simulink subsystem "OperatingModeAndErrorLogic"  (R2023b)
settings: Solver=VariableStepAuto  StartTime=0.0  StopTime=10  RelTol=1e-3
undefined symbols (not defined in the file): operatingMode
libraries: simulink x2
settings Model: DefaultTestHarness=Supervisory_Logic_Harness  Creator=vlenzi  LastModifiedBy=vlenzi

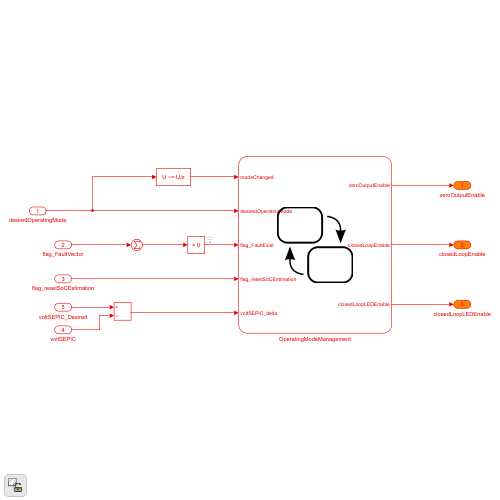
[thumbnail: Simulink's stored preview of the top-level diagram]
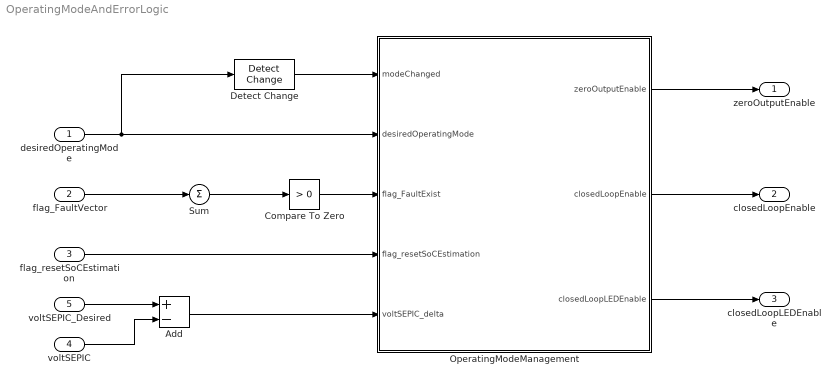
== system OperatingModeAndErrorLogic ==
  desiredOperatingMode : Inport
  flag_FaultVector : Inport  Port=2
  flag_resetSoCEstimation : Inport  Port=3
  voltSEPIC : Inport  Port=4
  voltSEPIC_Desired : Inport  Port=5
  Add : Sum  Inputs=+-
  Compare To Zero : simulink/Logic and Bit Operations/Compare To Zero  relop=>  OutDataTypeStr=boolean
  Detect Change : simulink/Logic and Bit Operations/Detect Change  vinit=operatingMode(0)  OutDataTypeStr=boolean
  OperatingModeManagement : Stateflow chart  TreatAsAtomicUnit=on
  Sum : Sum  Inputs=+
  zeroOutputEnable : Outport  OutDataTypeStr=boolean  Unit=1  PortDimensions=1
  closedLoopEnable : Outport  Port=2  OutDataTypeStr=boolean  Unit=1  PortDimensions=1
  closedLoopLEDEnable : Outport  Port=3  OutDataTypeStr=boolean  Unit=1  PortDimensions=1
  wires:
  Compare To Zero/1 -> OperatingModeManagement/3(flag_FaultExist)
  Sum/1 -> Compare To Zero/1
  OperatingModeManagement/3(closedLoopLEDEnable) -> closedLoopLEDEnable/1
  OperatingModeManagement/2(closedLoopEnable) -> closedLoopEnable/1
  flag_resetSoCEstimation/1 -> OperatingModeManagement/4(flag_resetSoCEstimation)
  OperatingModeManagement/1(zeroOutputEnable) -> zeroOutputEnable/1
  desiredOperatingMode/1 -> OperatingModeManagement/2(desiredOperatingMode), Detect Change/1
  Detect Change/1 -> OperatingModeManagement/1(modeChanged)
  flag_FaultVector/1 -> Sum/1
  voltSEPIC_Desired/1 -> Add/1
  voltSEPIC/1 -> Add/2
  Add/1 -> OperatingModeManagement/5(voltSEPIC_delta)

== stateflow chart OperatingModeAndErrorLogic/OperatingModeManagement ==
  state Operation
    state OperatingMode [parallel]
      settings: executionOrder=2
      state AllOpenLoop
        en:closedLoopEnable=false;
        en:closedLoopLEDEnable=false;
      state VoltOpen_CurrClosed
        en:closedLoopEnable=false;
        en:closedLoopLEDEnable=true;
      state VoltClosed_CurrOpen
        en:closedLoopEnable=true;
        en:closedLoopLEDEnable=false;
      state AllClosedLoop
        en:closedLoopEnable=true;
        en:closedLoopLEDEnable=true;
      state AutomaticOperation
        state AllOpenLoop
          en:closedLoopEnable=false;
          en:closedLoopLEDEnable=false;
        state WaitingForVoltageSettling
          en:closedLoopEnable=true;
          en:closedLoopLEDEnable=false;
        state AllClosedLoop
          en:closedLoopEnable=true;
          en:closedLoopLEDEnable=true;
        (default) -> Operation.OperatingMode.AutomaticOperation.AllOpenLoop
        Operation.OperatingMode.AutomaticOperation.AllOpenLoop -> WaitingForVoltageSettling : [abs(voltSEPIC_delta) <=1.5]
        WaitingForVoltageSettling -> Operation.OperatingMode.AutomaticOperation.AllOpenLoop [order 1] : [abs(voltSEPIC_delta) >2]
        WaitingForVoltageSettling -> Operation.OperatingMode.AutomaticOperation.AllClosedLoop [order 2] : [after(1,tick)]
      state NoOutput
        en:zeroOutputEnable=true;
      (default) -> (junction 91)
      (junction 91) -> Operation.OperatingMode.AllOpenLoop [order 1] : [desiredOperatingMode==AllOpenLoop]
      Operation.OperatingMode.AllOpenLoop -> OperatingMode : [modeChanged]
      (junction 91) -> (junction 92) [order 2]
      (junction 92) -> VoltOpen_CurrClosed [order 1] : [desiredOperatingMode==VoltOpen_CurrClosed]
      VoltOpen_CurrClosed -> OperatingMode : [modeChanged]
      (junction 92) -> (junction 93) [order 2]
      VoltClosed_CurrOpen -> OperatingMode : [modeChanged]
      (junction 93) -> VoltClosed_CurrOpen [order 1] : [desiredOperatingMode==VoltClosed_CurrOpen]
      (junction 93) -> (junction 94) [order 2]
      (junction 94) -> Operation.OperatingMode.AllClosedLoop [order 1] : [desiredOperatingMode==AllClosedLoop]
      Operation.OperatingMode.AllClosedLoop -> OperatingMode : [modeChanged]
      (junction 94) -> (junction 127) [order 2]
      (junction 127) -> AutomaticOperation [order 1] : [desiredOperatingMode==AutomaticOperation]
      (junction 127) -> NoOutput [order 2]
      AutomaticOperation -> OperatingMode : [modeChanged]
      NoOutput -> OperatingMode : [modeChanged]
    state CheckingFault [parallel]
      settings: executionOrder=1
      state SystemKO
        en:zeroOutputEnable=true;
      state SystemOK
        en:zeroOutputEnable=false;
      (default) -> SystemKO
      SystemOK -> SystemKO : [flag_FaultExist]
      SystemKO -> SystemOK : [~flag_FaultExist]
  state Initialization_no_output
    en:closedLoopEnable=false;
    en:closedLoopLEDEnable=false;
    en:zeroOutputEnable=true;
  (default) -> Initialization_no_output
  Initialization_no_output -> Operation : [desiredOperatingMode ~= NoOutput &&flag_resetSoCEstimation==0 ]
  data: modeChanged input boolean; zeroOutputEnable output boolean size=1; desiredOperatingMode input Enum: operatingMode; closedLoopEnable output boolean size=1; closedLoopLEDEnable output boolean size=1; flag_FaultExist input boolean; flag_resetSoCEstimation input boolean; voltSEPIC_delta input
